simulink model "wind_part"  (R2023b)
settings: Solver=VariableStepAuto  StartTime=0.0  StopTime=5  RelTol=1e-3
InitFcn:
  | Ld=0.3;
  | Lq=0.2;
  | Rs=2;
  | 
  | p=1;
  | Psi=0.2;
  | 
  | J=0.0005;
  | FF=0.0001;
  | 
  | KP_Id=1.28;
  | KI_Id=16.21;
  | KP_Iq=0.94;
  | KI_Iq=4.90;
  | 
  | KP_w=0.0784880455322167;
  | KI_w=0.0288211791619406;
  | 
  | f_pwm=1000;
  | Udc=50;
  | Ns=1;
  | Np=1;
  | R1=0.29;
  | C0=2100;
  | Cv=623;
  | R2=1.92;
  | C2=172;
  | 
  | %data_omega = load('max_CP_omega.mat');
  | 
  | %max_CP_omega = data_omega.max_CP_omega;
  | 
  | %max_CP_omega_param = Simulink.Parameter(max_CP_omega);
  | 
  | %max_CP_omega_param.CoderInfo.StorageClass = 'ExportedGlobal';
libraries: spsMosfetLib x6, simulink x6, slpidlib x4, spsCurrentMeasurementLib x4, spsSeriesRLCBranchLib x3, spsVoltageMeasurementLib x1, spsPermanentMagnetSynchronousMachineLib x1, spsdq0toabcLib x1, spsabctodq0Lib x1, spspowerguiLib x1
settings Model: Creator=hadek  LastModifiedBy=Peter
settings SolverCC: ZeroCrossAlgorithm=Adaptive  AlgebraicLoopSolver=TrustRegion
settings DataIOCC: SaveFormat=StructureWithTime  ReturnWorkspaceOutputs=off
settings DebuggingCC: IgnoredZcDiagnostic=none  UnconnectedInputMsg=warning  UnconnectedOutputMsg=warning  UnconnectedLineMsg=warning  ArithmeticOperatorsInVariantConditions=warning
settings ModelReferenceCC: EnableRefExpFcnMdlSchedulingChecks=on
settings SFSimCC: SimUseLocalCustomCode=off  CustomCodeUndefinedFunction=UseInterfaceOnly
settings RTWCC: RTWUseLocalCustomCode=off

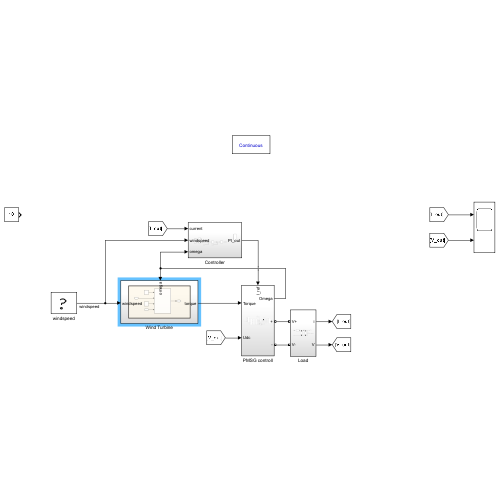
[thumbnail: Simulink's stored preview of the top-level diagram]
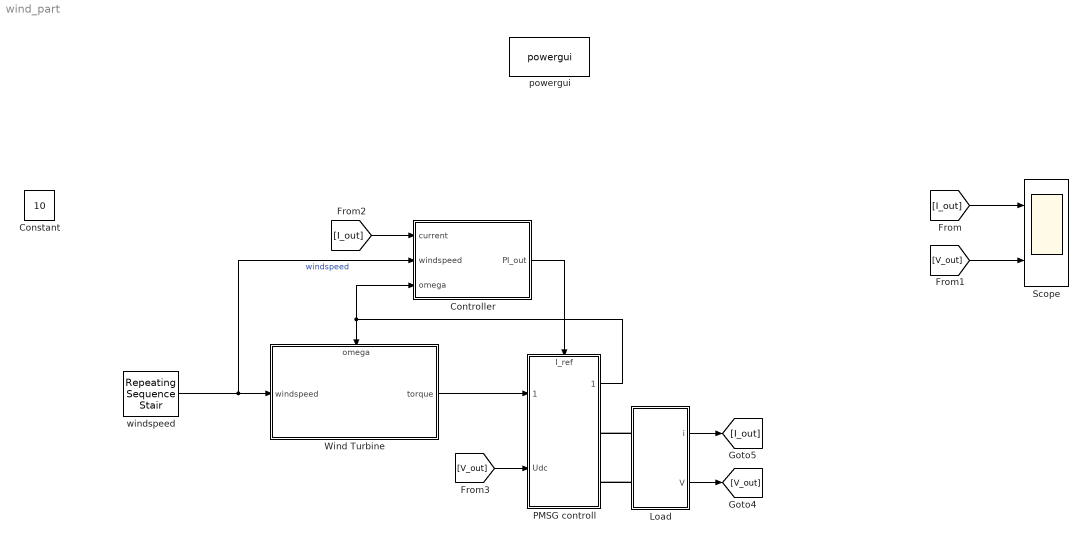
== system wind_part ==
  Constant : Constant  Value=10
  Controller : Subsystem
  Load : Subsystem
  PMSG controll : Subsystem
      settings: PortSchema="{\"entries\":[{\"content\":{\"sides\":[{\"content\":{\"connectorIds\":[\"In1\",\"In2\"]},\"type\":\"ConnectorPlacement.EquallySpacedRectSide\",\"uuid\":\"6ff45732-1fbe-44e6-bbf0-a97c0cfc251c\"},{\"content\":{\"connectorIds\":[\"Out1\",\"RConn1\",\"RConn2\"],\"side\":\"RIGHT\"},\"type\":\"ConnectorPlacement.EquallySpacedRectSide\",\"uuid\":\"615f7fbd-60ca-4bdf-8315-88a0e11d104a\"},{\"content\":{\"connectorIds\":[\"In3\"],\"side\":\"TOP\"},\"type\":\"ConnectorPlacement.EquallySpacedRectSide\",\"uuid\":\"73f43a16-ba4f-4676-a4ee-aa4b37dc4906\"}]},\"type\":\"ConnectorPlacement.EquallySpacedConnector\",\"uuid\":\"b405ac4b-096d-4645-a2b2-df92df1fd96d\"}],\"packageUris\":[\"http://schema.mathworks.com/mf0/Connector/R2020b\"],\"version\":\"1.0\"}"
  Scope : Scope  NumInputPorts=2
  Wind Turbine : Subsystem
      settings: PortSchema="{\"entries\":[{\"content\":{\"sides\":[{\"content\":{\"connectorIds\":[\"In1\"]},\"type\":\"ConnectorPlacement.EquallySpacedRectSide\",\"uuid\":\"d9607854-6c60-486c-bfea-e5bdfd6c8fa9\"},{\"content\":{\"connectorIds\":[\"Out1\"],\"side\":\"RIGHT\"},\"type\":\"ConnectorPlacement.EquallySpacedRectSide\",\"uuid\":\"5fa891cc-5ceb-404b-bebb-ba93c08d2f38\"},{\"content\":{\"connectorIds\":[\"In2\"],\"side\":\"TOP\"},\"type\":\"ConnectorPlacement.EquallySpacedRectSide\",\"uuid\":\"4840ec60-9cf6-480c-919e-88edc7040649\"}]},\"type\":\"ConnectorPlacement.EquallySpacedConnector\",\"uuid\":\"84375009-51d5-45f0-a301-b98d1305d1b8\"}],\"packageUris\":[\"http://schema.mathworks.com/mf0/Connector/R2020b\"],\"version\":\"1.0\"}"
  powergui : spspowerguiLib/powergui  Priority=1  SimulationMode=Continuous  SampleTime=50e-6  frequency=60  Iterations=50  frequencyindice=0  Pbase=100e6  ErrMax=1e-4  UnitsV=kV  UnitsW=MW  buscounter=0  FunctionMessages=off  echomessages=off  EnableUseOfTLC=off  CurrentSourceSwitches=off  DisableSnubberDevices=off  DisableRonSwitches=off  DisableVfSwitches=off  DisplayEquations=off  AutomaticDiscreteSolvers=off  SolverType=Tustin/Backward Euler (TBE)  Interpol=off  ExternalGateDelay=off  methode=off  Ts=100  x0status=blocks  SPID=on  SwTol=0  HookPort=off  NonlinearTolerance=1e-4  nMaxIteration=100  ContinueOnMaxIteration=off  RestoreLinks=warning  ResistiveCurrentMeasurement=off  Frange=[0:2:500]  Ylog=off  Xlog=on  ShowGrid=off  save=off  variable=ZData  structure=0  ZoomFFT=off  StartTime=0.0  cycles=1  DisplayStyle=1  fundamental=60  FreqAxis=off  MaxFrequency=1000  frequencyindicesteady=1  RmsSteady=1  display=off
  windspeed : simulink/Sources/Repeating Sequence Stair  OutValues=windspeed  tsamp=0.2  OutMin=[]  OutMax=[]  OutDataTypeStr=double  OutputDataTypeScalingMode=double  OutDataType=fixdt(0,8)  ConRadixGroup=Best Precision: Vector-wise  OutScaling=2^-12
  wires:
  Load/1(i) -> [I_out]
  Load/2(V) -> [V_out]
  Wind Turbine/1(torque) -> PMSG controll/1(Torque)
  [I_out] -> Scope/1
  [V_out] -> Scope/2
  PMSG controll/1(Omega) -> Controller/3(omega), Wind Turbine/2(omega)
  Controller/1(PI_out) -> PMSG controll/3(I_ref)
  [I_out] -> Controller/1(current)
  [V_out] -> PMSG controll/2(Udc)
  windspeed/1 -> Wind Turbine/1(windspeed), Controller/2(windspeed)  "windspeed"
  connections:
  Load/LConn1 -- PMSG controll/RConn1
  Load/LConn2 -- PMSG controll/RConn2

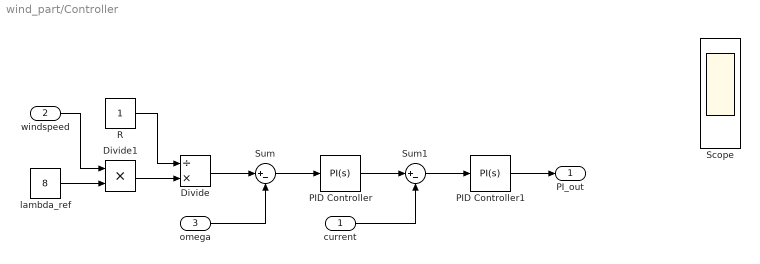
== system wind_part/Controller ==
  current : Inport
  windspeed : Inport  Port=2
  omega : Inport  Port=3
  Divide : Product  Inputs=/*
  Divide1 : Product  Inputs=**
  PID Controller : slpidlib/PID Controller  Controller=PI  Form=Parallel  TimeDomain=Continuous-time  UseExternalTs=off  SampleTime=-1  IntegratorMethod=Forward Euler  FilterMethod=Forward Euler  ControllerParametersSource=internal  P=1  I=1  UseKiTs=off  D=0  N=100  UseFilter=on  TunerSelectOption=Transfer Function Based (PID Tuner App)  InitialConditionSource=internal  InitialConditionForIntegrator=0  InitialConditionForFilter=0  DifferentiatorICPrevScaledInput=0  ExternalReset=none  TrackingMode=off  Kt=1  LimitOutput=off  SatLimitsSource=internal  UpperSaturationLimit=20  LowerSaturationLimit=-20  LinearizeAsGain=on  AntiWindupMode=none  Kb=1  LimitIntegrator=off  UpperIntegratorSaturationLimit=inf  LowerIntegratorSaturationLimit=-inf  POutMin=[]  POutMax=[]  IOutMin=[]  IOutMax=[]  DOutMin=[]  DOutMax=[]  NOutMin=[]  NOutMax=[]  SumOutMin=[]  SumOutMax=[]  SaturationOutMin=[]  SaturationOutMax=[]  PParamMin=[]  PParamMax=[]  IParamMin=[]  IParamMax=[]  DParamMin=[]  DParamMax=[]  NParamMin=[]  NParamMax=[]  KbParamMin=[]  KbParamMax=[]  KtParamMin=[]  KtParamMax=[]  KbOutMin=[]  KbOutMax=[]  KtOutMin=[]  KtOutMax=[]  IntegratorOutMin=[]  IntegratorOutMax=[]  FilterOutMin=[]  FilterOutMax=[]  SumI1OutMin=[]  SumI1OutMax=[]  SumI2OutMin=[]  SumI2OutMax=[]  SumI3OutMin=[]  SumI3OutMax=[]  SumI4OutMin=[]  SumI4OutMax=[]  SumDOutMin=[]  SumDOutMax=[]  DifferentiatorOutMin=[]  DifferentiatorOutMax=[]  FilterDiffOutCoefMin=[]  FilterDiffOutCoefMax=[]  ReciprocalOutMin=[]  ReciprocalOutMax=[]  SumDenOutMin=[]  SumDenOutMax=[]  SumNumOutMin=[]  SumNumOutMax=[]  DivideOutMin=[]  DivideOutMax=[]  UdiffTsProdOutMin=[]  UdiffTsProdOutMax=[]  NTsProdOutMin=[]  NTsProdOutMax=[]  UintegralTsProdOutMin=[]  UintegralTsProdOutMax=[]  UngainTsProdOutMin=[]  UngainTsProdOutMax=[]  ClampingZeroOutDataTypeStr=Inherit: Inherit via back propagation  ClampingZeroOutMin=[]  ClampingZeroOutMax=[]  FilterDenConstantOutDataTypeStr=Inherit: Inherit via back propagation  FilterDenConstantOutMin=[]  FilterDenConstantOutMax=[]  PCopyOutDataTypeStr=Inherit: Inherit via back propagation  PCopyOutMin=[]  PCopyOutMax=[]  NCopyOutDataTypeStr=Inherit: Inherit via back propagation  NCopyOutMin=[]  NCopyOutMax=[]  IntegratorContinuousStateAttributes=''  IntegratorStateMustResolveToSignalObject=off  IntegratorRTWStateStorageClass=Auto  FilterContinuousStateAttributes=''  FilterStateMustResolveToSignalObject=off  FilterRTWStateStorageClass=Auto  ParallelPVariant=InternalParameters  IdealPVariant=Disabled  IVariant=InternalParameters  DVariant=Disabled  IntegratorVariant=Continuous  SatVariant=Disabled  AWVariant=Passthrough  PCopyVariant=Disabled  TRVariant=Disabled  FdbkBlocksVariant=Forward  IdealPFdbkVariant=Disabled  SatFdbkVariant=Disabled  DerivativeFilterVariant=Disabled  NVariant=Disabled  NCopyVariant=Disabled_SignalSpec  FilterICVariant=Disabled  IntegratorICVariant=InternalICs  ExternalResetVariant=Disabled  TRSumVariant=Passthrough  SumFdbkVariant=Disabled  SumVariant=Sum_PI  TsampFilterVariant=InternalTs  TsampNgainVariant=Passthrough  TsampIntegralVariant=Disabled_SignalSpec  ExternalSaturationOutDataTypeStr=Inherit: Same as second input
  PID Controller1 : slpidlib/PID Controller  Controller=PI  Form=Parallel  TimeDomain=Continuous-time  UseExternalTs=off  SampleTime=-1  IntegratorMethod=Forward Euler  FilterMethod=Forward Euler  ControllerParametersSource=internal  P=1  I=1  UseKiTs=off  D=0  N=100  UseFilter=on  TunerSelectOption=Transfer Function Based (PID Tuner App)  InitialConditionSource=internal  InitialConditionForIntegrator=0  InitialConditionForFilter=0  DifferentiatorICPrevScaledInput=0  ExternalReset=none  TrackingMode=off  Kt=1  LimitOutput=off  SatLimitsSource=internal  UpperSaturationLimit=20  LowerSaturationLimit=-20  LinearizeAsGain=on  AntiWindupMode=none  Kb=1  LimitIntegrator=off  UpperIntegratorSaturationLimit=inf  LowerIntegratorSaturationLimit=-inf  POutMin=[]  POutMax=[]  IOutMin=[]  IOutMax=[]  DOutMin=[]  DOutMax=[]  NOutMin=[]  NOutMax=[]  SumOutMin=[]  SumOutMax=[]  SaturationOutMin=[]  SaturationOutMax=[]  PParamMin=[]  PParamMax=[]  IParamMin=[]  IParamMax=[]  DParamMin=[]  DParamMax=[]  NParamMin=[]  NParamMax=[]  KbParamMin=[]  KbParamMax=[]  KtParamMin=[]  KtParamMax=[]  KbOutMin=[]  KbOutMax=[]  KtOutMin=[]  KtOutMax=[]  IntegratorOutMin=[]  IntegratorOutMax=[]  FilterOutMin=[]  FilterOutMax=[]  SumI1OutMin=[]  SumI1OutMax=[]  SumI2OutMin=[]  SumI2OutMax=[]  SumI3OutMin=[]  SumI3OutMax=[]  SumI4OutMin=[]  SumI4OutMax=[]  SumDOutMin=[]  SumDOutMax=[]  DifferentiatorOutMin=[]  DifferentiatorOutMax=[]  FilterDiffOutCoefMin=[]  FilterDiffOutCoefMax=[]  ReciprocalOutMin=[]  ReciprocalOutMax=[]  SumDenOutMin=[]  SumDenOutMax=[]  SumNumOutMin=[]  SumNumOutMax=[]  DivideOutMin=[]  DivideOutMax=[]  UdiffTsProdOutMin=[]  UdiffTsProdOutMax=[]  NTsProdOutMin=[]  NTsProdOutMax=[]  UintegralTsProdOutMin=[]  UintegralTsProdOutMax=[]  UngainTsProdOutMin=[]  UngainTsProdOutMax=[]  ClampingZeroOutDataTypeStr=Inherit: Inherit via back propagation  ClampingZeroOutMin=[]  ClampingZeroOutMax=[]  FilterDenConstantOutDataTypeStr=Inherit: Inherit via back propagation  FilterDenConstantOutMin=[]  FilterDenConstantOutMax=[]  PCopyOutDataTypeStr=Inherit: Inherit via back propagation  PCopyOutMin=[]  PCopyOutMax=[]  NCopyOutDataTypeStr=Inherit: Inherit via back propagation  NCopyOutMin=[]  NCopyOutMax=[]  IntegratorContinuousStateAttributes=''  IntegratorStateMustResolveToSignalObject=off  IntegratorRTWStateStorageClass=Auto  FilterContinuousStateAttributes=''  FilterStateMustResolveToSignalObject=off  FilterRTWStateStorageClass=Auto  ParallelPVariant=InternalParameters  IdealPVariant=Disabled  IVariant=InternalParameters  DVariant=Disabled  IntegratorVariant=Continuous  SatVariant=Disabled  AWVariant=Passthrough  PCopyVariant=Disabled  TRVariant=Disabled  FdbkBlocksVariant=Forward  IdealPFdbkVariant=Disabled  SatFdbkVariant=Disabled  DerivativeFilterVariant=Disabled  NVariant=Disabled  NCopyVariant=Disabled_SignalSpec  FilterICVariant=Disabled  IntegratorICVariant=InternalICs  ExternalResetVariant=Disabled  TRSumVariant=Passthrough  SumFdbkVariant=Disabled  SumVariant=Sum_PI  TsampFilterVariant=InternalTs  TsampNgainVariant=Passthrough  TsampIntegralVariant=Disabled_SignalSpec  ExternalSaturationOutDataTypeStr=Inherit: Same as second input
  R : Constant
  Scope : Scope  NumInputPorts=5
  Sum : Sum  Inputs=|+-
  Sum1 : Sum  Inputs=|+-
  lambda_ref : Constant  Value=8
  PI_out : Outport
  wires:
  R/1 -> Divide/1
  lambda_ref/1 -> Divide1/2
  Divide1/1 -> Divide/2
  windspeed/1 -> Divide1/1
  Sum/1 -> PID Controller/1
  Divide/1 -> Sum/1
  Sum1/1 -> PID Controller1/1
  PID Controller1/1 -> PI_out/1
  PID Controller/1 -> Sum1/1
  current/1 -> Sum1/2
  omega/1 -> Sum/2

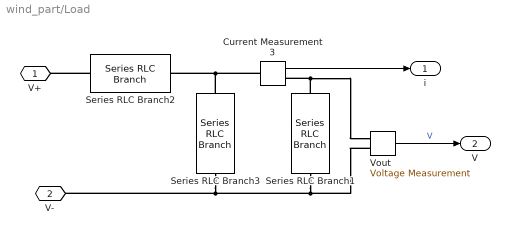
== system wind_part/Load ==
  " Vout" : spsVoltageMeasurementLib/Voltage Measurement  PhasorSimulation=off  OutputType=Complex  PSBequivalent=0
  Current Measurement3 : spsCurrentMeasurementLib/Current Measurement  PhasorSimulation=off  OutputType=Complex  PSBequivalent=0
  Series RLC Branch1 : spsSeriesRLCBranchLib/Series RLC Branch  LConnTagsString=__new0  RConnTagsString=__new0  BranchType=R  Resistance=10  Inductance=1e-3  SetiL0=off  InitialCurrent=0  Capacitance=2e-3  Setx0=off  InitialVoltage=0  Measurements=None
  Series RLC Branch2 : spsSeriesRLCBranchLib/Series RLC Branch  LConnTagsString=__new0  RConnTagsString=__new0  BranchType=L  Resistance=10  Inductance=100e-3  SetiL0=off  InitialCurrent=0  Capacitance=2e-3  Setx0=off  InitialVoltage=0  Measurements=None
  Series RLC Branch3 : spsSeriesRLCBranchLib/Series RLC Branch  LConnTagsString=__new0  RConnTagsString=__new0  BranchType=C  Resistance=10  Inductance=1e-3  SetiL0=off  InitialCurrent=0  Capacitance=2e-3  Setx0=on  InitialVoltage=50  Measurements=None
  V+ : PMIOPort  Side=Left
  V- : PMIOPort  Port=2  Side=Left
  i : Outport
  V : Outport  Port=2
  wires:
  " Vout"/1 -> V/1  "V"
  Current Measurement3/1 -> i/1
  connections:
  Series RLC Branch3/LConn1 -- Current Measurement3/LConn1 -- Series RLC Branch2/RConn1
  Current Measurement3/RConn1 -- Series RLC Branch1/LConn1 -- " Vout"/LConn1
  Series RLC Branch3/RConn1 -- " Vout"/LConn2 -- Series RLC Branch1/RConn1 -- V-/RConn1
  Series RLC Branch2/LConn1 -- V+/RConn1

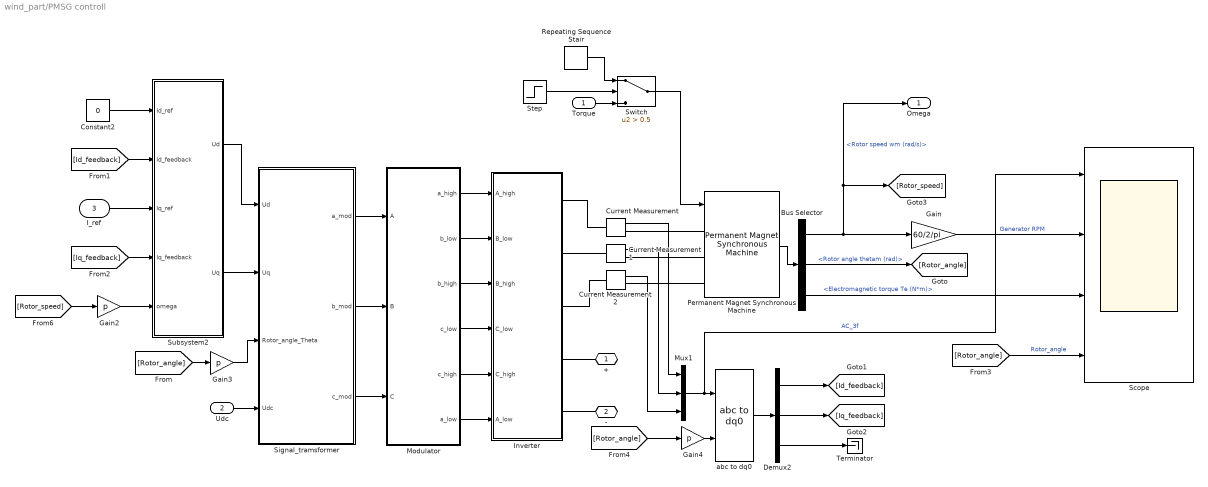
== system wind_part/PMSG controll ==
  Torque : Inport
  Udc : Inport  Port=2
  I_ref : Inport  Port=3
  Bus Selector : BusSelector  OutputSignals=Rotor speed wm (rad/s),Rotor angle thetam (rad),Electromagnetic torque Te (N*m)
  Constant2 : Constant  Value=0
  Current Measurement : spsCurrentMeasurementLib/Current Measurement  PhasorSimulation=off  OutputType=Complex  PSBequivalent=0
  Current Measurement1 : spsCurrentMeasurementLib/Current Measurement  PhasorSimulation=off  OutputType=Complex  PSBequivalent=0
  Current Measurement2 : spsCurrentMeasurementLib/Current Measurement  PhasorSimulation=off  OutputType=Complex  PSBequivalent=0
  Demux2 : Demux  Outputs=3
  Gain : Gain  Gain=60/2/pi
  Gain2 : Gain  Gain=p
  Gain3 : Gain  Gain=p
  Gain4 : Gain  Gain=p
  Inverter : Subsystem
  Modulator : Subsystem
  Mux1 : Mux  Inputs=3
  Permanent Magnet Synchronous Machine : spsPermanentMagnetSynchronousMachineLib/Permanent Magnet Synchronous Machine  NbPhases=3  FluxDistribution=Sinusoidal  RotorType=Salient-pole  MechanicalLoad=Torque Tm  PresetModel=No  ShowDetailedParameters=on  MeasurementBus=off  Resistance=Rs  Inductance=8.5e-3  dqInductances=[Ld,Lq]  La=0.000395  MachineConstant=Flux linkage established by magnets (V.s)  Flux=Psi  VoltageCst=36.276  TorqueCst=0.3  Flat=120  Mechanical=[J FF p 0]  PolePairs=4  InitialConditions=[0,0, 0,0]  InitialConditions5ph=[0 0 0 0 0 0]  RefAngle=90 degrees behind phase A axis (modified Park)  IterativeDiscreteModel=Trapezoidal non iterative  TsBlock=-1  TsPowergui=0
  Repeating Sequence Stair : simulink/Sources/Repeating Sequence Stair  OutValues=0.1:0.1:5  tsamp=0.02  OutMin=[]  OutMax=[]  OutDataTypeStr=double  OutputDataTypeScalingMode=double  OutDataType=fixdt(0,8)  ConRadixGroup=Best Precision: Vector-wise  OutScaling=2^-12
  Scope : Scope  NumInputPorts=4
  Signal_tramsformer : Subsystem
  Step : Step  Time=5  Before=1  After=0  SampleTime=0
  Subsystem2 : Subsystem
  Switch : Switch  Criteria=u2 > Threshold  Threshold=0.5  SaturateOnIntegerOverflow=off  InputSameDT=off
  Terminator : Terminator
  abc to dq0 : spsabctodq0Lib/abc to dq0  Alignment=90 degrees behind phase A axis
  + : PMIOPort  Side=Right
  - : PMIOPort  Port=2  Side=Right
  Omega : Outport
  wires:
  Current Measurement/1 -> Mux1/1
  [Rotor_speed] -> Gain2/1
  [Rotor_angle] -> Gain4/1
  Current Measurement2/1 -> Mux1/3
  [Rotor_angle] -> Gain3/1
  Subsystem2/2(Uq) -> Signal_tramsformer/2(Uq)
  Demux2/2 -> [Iq_feedback]
  Bus Selector/1 -> [Rotor_speed], Omega/1, Gain/1  "<Rotor speed wm (rad/s)>"
  [Id_feedback] -> Subsystem2/2(Id_feedback)
  Signal_tramsformer/3(c_mod) -> Modulator/3(C)
  Bus Selector/3 -> Scope/3  "<Electromagnetic torque Te (N*m)>"
  Bus Selector/2 -> [Rotor_angle]  "<Rotor angle thetam (rad)>"
  abc to dq0/1 -> Demux2/1
  Demux2/1 -> [Id_feedback]
  Signal_tramsformer/2(b_mod) -> Modulator/2(B)
  Constant2/1 -> Subsystem2/1(Id_ref)
  Mux1/1 -> Scope/1, abc to dq0/1  "AC_3f"
  Demux2/3 -> Terminator/1
  Current Measurement1/1 -> Mux1/2
  [Iq_feedback] -> Subsystem2/4(Iq_feedback)
  Gain/1 -> Scope/2  "Generator RPM"
  Signal_tramsformer/1(a_mod) -> Modulator/1(A)
  I_ref/1 -> Subsystem2/3(Iq_ref)
  Subsystem2/1(Ud) -> Signal_tramsformer/1(Ud)
  [Rotor_angle] -> Scope/4  "Rotor_angle"
  Permanent Magnet Synchronous Machine/1 -> Bus Selector/1
  Gain4/1 -> abc to dq0/2
  Gain3/1 -> Signal_tramsformer/3(Rotor_angle_Theta)
  Gain2/1 -> Subsystem2/5(omega)
  Torque/1 -> Switch/3
  Udc/1 -> Signal_tramsformer/4(Udc)
  Modulator/5(c_high) -> Inverter/5(C_high)
  Modulator/6(a_low) -> Inverter/6(A_low)
  Modulator/4(c_low) -> Inverter/4(C_low)
  Modulator/2(b_low) -> Inverter/2(B_low)
  Modulator/1(a_high) -> Inverter/1(A_high)
  Modulator/3(b_high) -> Inverter/3(" B_high")
  Step/1 -> Switch/2
  Switch/1 -> Permanent Magnet Synchronous Machine/1
  Repeating Sequence Stair/1 -> Switch/1
  connections:
  Current Measurement2/RConn1 -- Permanent Magnet Synchronous Machine/LConn3
  Current Measurement1/RConn1 -- Permanent Magnet Synchronous Machine/LConn2
  Inverter/RConn3 -- Current Measurement2/LConn1
  Inverter/RConn1 -- Current Measurement/LConn1
  Inverter/RConn2 -- Current Measurement1/LConn1
  Permanent Magnet Synchronous Machine/LConn1 -- Current Measurement/RConn1
  Inverter/RConn5 -- -/RConn1
  Inverter/RConn4 -- +/RConn1

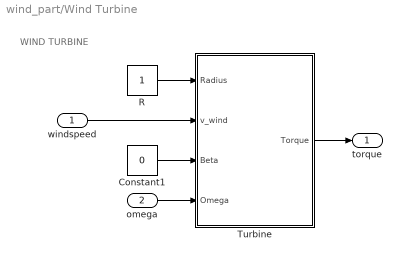
== system wind_part/Wind Turbine ==
  note: WIND TURBINE
  windspeed : Inport
  omega : Inport  Port=2
  Constant1 : Constant  Value=0
  R : Constant
  Turbine : Subsystem
  torque : Outport
  wires:
  R/1 -> Turbine/1(Radius)
  omega/1 -> Turbine/4(Omega)
  Constant1/1 -> Turbine/3(Beta)
  windspeed/1 -> Turbine/2(v_wind)
  Turbine/1(Torque) -> torque/1

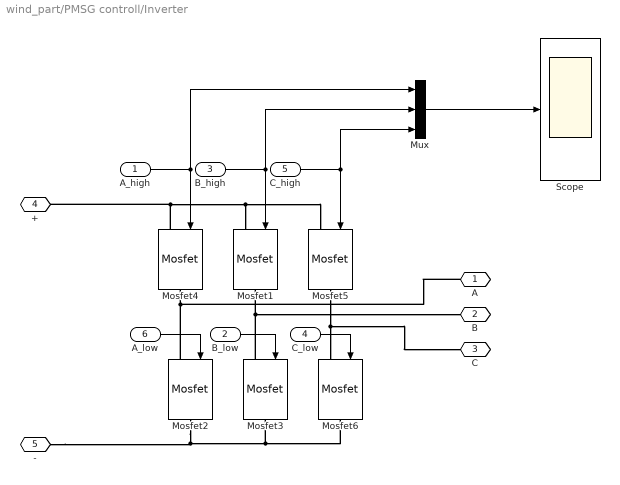
== system wind_part/PMSG controll/Inverter ==
  A_high : Inport
  B_low : Inport  Port=2
  " B_high" : Inport  Port=3
  C_low : Inport  Port=4
  C_high : Inport  Port=5
  A_low : Inport  Port=6
  Mosfet{1..6} (6 alike) : spsMosfetLib/Mosfet  Ron=0.1  Lon=0  Rd=0.01  Vfd=0  IC=0  Rs=1e5  Cs=inf  Measurements=off
  Mux : Mux  Inputs=3
  Scope : Scope
  A : PMIOPort  Side=Right
  B : PMIOPort  Port=2  Side=Right
  C : PMIOPort  Port=3  Side=Right
  + : PMIOPort  Port=4  Side=Right
  - : PMIOPort  Port=5  Side=Right
  wires:
  A_high/1 -> Mux/1, Mosfet4/1
  C_high/1 -> Mux/3, Mosfet5/1
  " B_high"/1 -> Mux/2, Mosfet1/1
  Mux/1 -> Scope/1
  B_low/1 -> Mosfet3/1
  C_low/1 -> Mosfet6/1
  A_low/1 -> Mosfet2/1
  connections:
  Mosfet4/LConn1 -- +/RConn1 -- Mosfet5/LConn1 -- Mosfet1/LConn1
  Mosfet5/RConn1 -- Mosfet6/LConn1 -- C/RConn1
  Mosfet3/LConn1 -- B/RConn1 -- Mosfet1/RConn1
  Mosfet2/RConn1 -- -/RConn1 -- Mosfet6/RConn1 -- Mosfet3/RConn1
  Mosfet2/LConn1 -- A/RConn1 -- Mosfet4/RConn1

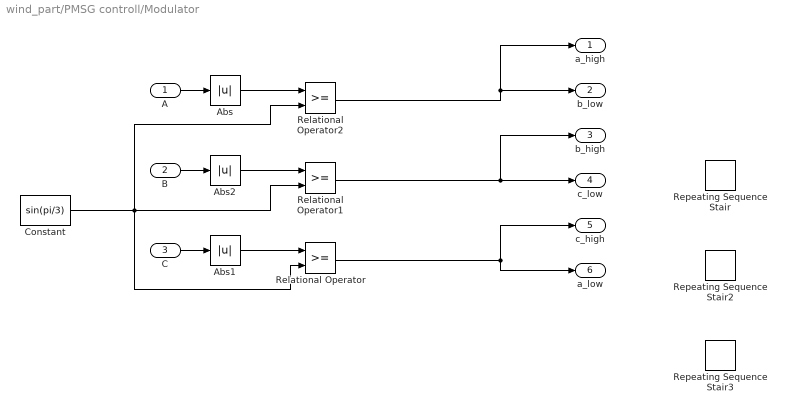
== system wind_part/PMSG controll/Modulator ==
  A : Inport
  B : Inport  Port=2
  C : Inport  Port=3
  Abs : Abs  SaturateOnIntegerOverflow=off
  Abs1 : Abs  SaturateOnIntegerOverflow=off
  Abs2 : Abs  SaturateOnIntegerOverflow=off
  Constant : Constant  Value=sin(pi/3)
  Relational Operator : RelationalOperator  OutDataTypeStr=boolean  RndMeth=Simplest  InputSameDT=off
  Relational Operator1 : RelationalOperator  OutDataTypeStr=boolean  RndMeth=Simplest  InputSameDT=off
  Relational Operator2 : RelationalOperator  OutDataTypeStr=boolean  RndMeth=Simplest  InputSameDT=off
  Repeating Sequence Stair : simulink/Sources/Repeating Sequence Stair  OutValues=[0 1 1 0 0 0 0 1 1 0 0 0]  tsamp=30/(360)  OutMin=[]  OutMax=[]  OutDataTypeStr=double  OutputDataTypeScalingMode=double  OutDataType=fixdt(0,8)  ConRadixGroup=Best Precision: Vector-wise  OutScaling=2^-12
  Repeating Sequence Stair2 : simulink/Sources/Repeating Sequence Stair  OutValues=[1 0 0 0 0 1 1 0 0 0 0 1]  tsamp=30/360  OutMin=[]  OutMax=[]  OutDataTypeStr=double  OutputDataTypeScalingMode=double  OutDataType=fixdt(0,8)  ConRadixGroup=Best Precision: Vector-wise  OutScaling=2^-12
  Repeating Sequence Stair3 : simulink/Sources/Repeating Sequence Stair  OutValues=[0 0 0 1 1 0 0 0 0 1 1 0]  tsamp=30/360  OutMin=[]  OutMax=[]  OutDataTypeStr=double  OutputDataTypeScalingMode=double  OutDataType=fixdt(0,8)  ConRadixGroup=Best Precision: Vector-wise  OutScaling=2^-12
  a_high : Outport
  b_low : Outport  Port=2
  b_high : Outport  Port=3
  c_low : Outport  Port=4
  c_high : Outport  Port=5
  a_low : Outport  Port=6
  wires:
  B/1 -> Abs2/1
  C/1 -> Abs1/1
  A/1 -> Abs/1
  Relational Operator2/1 -> a_high/1, b_low/1
  Relational Operator1/1 -> b_high/1, c_low/1
  Relational Operator/1 -> c_high/1, a_low/1
  Constant/1 -> Relational Operator2/2, Relational Operator1/2, Relational Operator/2
  Abs/1 -> Relational Operator2/1
  Abs1/1 -> Relational Operator/1
  Abs2/1 -> Relational Operator1/1

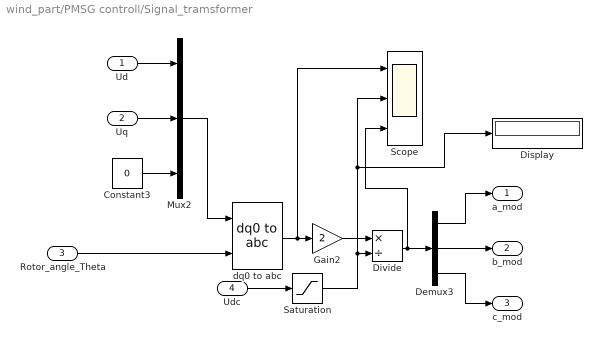
== system wind_part/PMSG controll/Signal_tramsformer ==
  Ud : Inport
  Uq : Inport  Port=2
  Rotor_angle_Theta : Inport  Port=3
  Udc : Inport  Port=4
  Constant3 : Constant  Value=0
  Demux3 : Demux  Outputs=3
  Display : Display
  Divide : Product  Inputs=*/
  Gain2 : Gain  Gain=2
  Mux2 : Mux  Inputs=3
  Saturation : Saturate  UpperLimit=inf  LowerLimit=1e-1
  Scope : Scope  NumInputPorts=3
  dq0 to abc : spsdq0toabcLib/dq0 to abc  Alignment=90 degrees behind phase A axis
  a_mod : Outport
  b_mod : Outport  Port=2
  c_mod : Outport  Port=3
  wires:
  Demux3/1 -> a_mod/1
  Udc/1 -> Saturation/1
  Divide/1 -> Scope/3, Demux3/1
  dq0 to abc/1 -> Scope/1, Gain2/1
  Gain2/1 -> Divide/1
  Mux2/1 -> dq0 to abc/1
  Constant3/1 -> Mux2/3
  Demux3/3 -> c_mod/1
  Demux3/2 -> b_mod/1
  Ud/1 -> Mux2/1
  Uq/1 -> Mux2/2
  Rotor_angle_Theta/1 -> dq0 to abc/2
  Saturation/1 -> Scope/2, Display/1, Divide/2

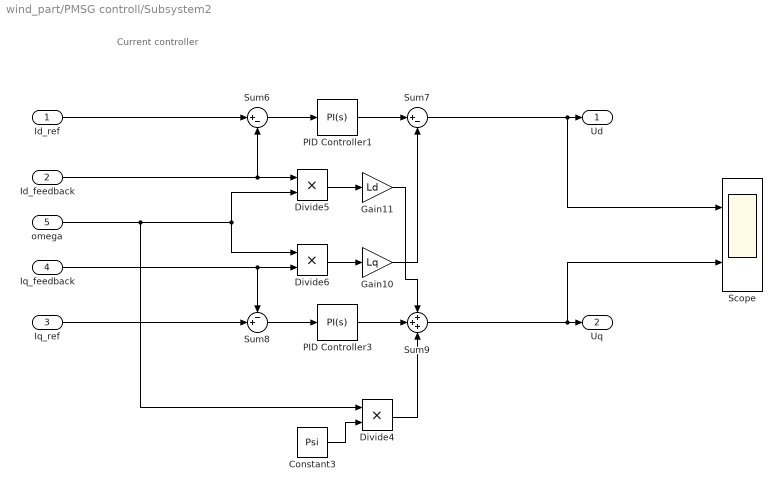
== system wind_part/PMSG controll/Subsystem2 ==
  note: Current controller
  Id_ref : Inport
  Id_feedback : Inport  Port=2
  Iq_ref : Inport  Port=3
  Iq_feedback : Inport  Port=4
  omega : Inport  Port=5
  Constant3 : Constant  Value=Psi
  Divide4 : Product  Inputs=**
  Divide5 : Product  Inputs=**
  Divide6 : Product  Inputs=**
  Gain10 : Gain  Gain=Lq
  Gain11 : Gain  Gain=Ld
  PID Controller1 : slpidlib/PID Controller  Controller=PI  Form=Parallel  TimeDomain=Continuous-time  UseExternalTs=off  SampleTime=-1  IntegratorMethod=Forward Euler  FilterMethod=Forward Euler  ControllerParametersSource=internal  P=KP_Id  I=KI_Id  UseKiTs=off  D=0  N=100  UseFilter=on  TunerSelectOption=Transfer Function Based (PID Tuner App)  InitialConditionSource=internal  InitialConditionForIntegrator=0  InitialConditionForFilter=0  DifferentiatorICPrevScaledInput=0  ExternalReset=none  TrackingMode=off  Kt=1  LimitOutput=off  SatLimitsSource=internal  UpperSaturationLimit=650  LowerSaturationLimit=-650  LinearizeAsGain=on  AntiWindupMode=none  Kb=1  LimitIntegrator=off  UpperIntegratorSaturationLimit=inf  LowerIntegratorSaturationLimit=-inf  POutMin=[]  POutMax=[]  IOutMin=[]  IOutMax=[]  DOutMin=[]  DOutMax=[]  NOutMin=[]  NOutMax=[]  SumOutMin=[]  SumOutMax=[]  SaturationOutMin=[]  SaturationOutMax=[]  PParamMin=[]  PParamMax=[]  IParamMin=[]  IParamMax=[]  DParamMin=[]  DParamMax=[]  NParamMin=[]  NParamMax=[]  KbParamMin=[]  KbParamMax=[]  KtParamMin=[]  KtParamMax=[]  KbOutMin=[]  KbOutMax=[]  KtOutMin=[]  KtOutMax=[]  IntegratorOutMin=[]  IntegratorOutMax=[]  FilterOutMin=[]  FilterOutMax=[]  SumI1OutMin=[]  SumI1OutMax=[]  SumI2OutMin=[]  SumI2OutMax=[]  SumI3OutMin=[]  SumI3OutMax=[]  SumI4OutMin=[]  SumI4OutMax=[]  SumDOutMin=[]  SumDOutMax=[]  DifferentiatorOutMin=[]  DifferentiatorOutMax=[]  FilterDiffOutCoefMin=[]  FilterDiffOutCoefMax=[]  ReciprocalOutMin=[]  ReciprocalOutMax=[]  SumDenOutMin=[]  SumDenOutMax=[]  SumNumOutMin=[]  SumNumOutMax=[]  DivideOutMin=[]  DivideOutMax=[]  UdiffTsProdOutMin=[]  UdiffTsProdOutMax=[]  NTsProdOutMin=[]  NTsProdOutMax=[]  UintegralTsProdOutMin=[]  UintegralTsProdOutMax=[]  UngainTsProdOutMin=[]  UngainTsProdOutMax=[]  ClampingZeroOutDataTypeStr=Inherit: Inherit via back propagation  ClampingZeroOutMin=[]  ClampingZeroOutMax=[]  FilterDenConstantOutDataTypeStr=Inherit: Inherit via back propagation  FilterDenConstantOutMin=[]  FilterDenConstantOutMax=[]  PCopyOutDataTypeStr=Inherit: Inherit via back propagation  PCopyOutMin=[]  PCopyOutMax=[]  NCopyOutDataTypeStr=Inherit: Inherit via back propagation  NCopyOutMin=[]  NCopyOutMax=[]  IntegratorContinuousStateAttributes=''  IntegratorStateMustResolveToSignalObject=off  IntegratorRTWStateStorageClass=Auto  FilterContinuousStateAttributes=''  FilterStateMustResolveToSignalObject=off  FilterRTWStateStorageClass=Auto  ParallelPVariant=InternalParameters  IdealPVariant=Disabled  IVariant=InternalParameters  DVariant=Disabled  IntegratorVariant=Continuous  SatVariant=Disabled  AWVariant=Passthrough  PCopyVariant=Disabled  TRVariant=Disabled  FdbkBlocksVariant=Forward  IdealPFdbkVariant=Disabled  SatFdbkVariant=Disabled  DerivativeFilterVariant=Disabled  NVariant=Disabled  NCopyVariant=Disabled_SignalSpec  FilterICVariant=Disabled  IntegratorICVariant=InternalICs  ExternalResetVariant=Disabled  TRSumVariant=Passthrough  SumFdbkVariant=Disabled  SumVariant=Sum_PI  TsampFilterVariant=InternalTs  TsampNgainVariant=Passthrough  TsampIntegralVariant=Disabled_SignalSpec  ExternalSaturationOutDataTypeStr=Inherit: Same as second input
  PID Controller3 : slpidlib/PID Controller  Controller=PI  Form=Parallel  TimeDomain=Continuous-time  UseExternalTs=off  SampleTime=-1  IntegratorMethod=Forward Euler  FilterMethod=Forward Euler  ControllerParametersSource=internal  P=KP_Iq  I=KI_Iq  UseKiTs=off  D=0  N=100  UseFilter=on  TunerSelectOption=Transfer Function Based (PID Tuner App)  InitialConditionSource=internal  InitialConditionForIntegrator=0  InitialConditionForFilter=0  DifferentiatorICPrevScaledInput=0  ExternalReset=none  TrackingMode=off  Kt=1  LimitOutput=off  SatLimitsSource=internal  UpperSaturationLimit=650  LowerSaturationLimit=-650  LinearizeAsGain=on  AntiWindupMode=none  Kb=1  LimitIntegrator=off  UpperIntegratorSaturationLimit=inf  LowerIntegratorSaturationLimit=-inf  POutMin=[]  POutMax=[]  IOutMin=[]  IOutMax=[]  DOutMin=[]  DOutMax=[]  NOutMin=[]  NOutMax=[]  SumOutMin=[]  SumOutMax=[]  SaturationOutMin=[]  SaturationOutMax=[]  PParamMin=[]  PParamMax=[]  IParamMin=[]  IParamMax=[]  DParamMin=[]  DParamMax=[]  NParamMin=[]  NParamMax=[]  KbParamMin=[]  KbParamMax=[]  KtParamMin=[]  KtParamMax=[]  KbOutMin=[]  KbOutMax=[]  KtOutMin=[]  KtOutMax=[]  IntegratorOutMin=[]  IntegratorOutMax=[]  FilterOutMin=[]  FilterOutMax=[]  SumI1OutMin=[]  SumI1OutMax=[]  SumI2OutMin=[]  SumI2OutMax=[]  SumI3OutMin=[]  SumI3OutMax=[]  SumI4OutMin=[]  SumI4OutMax=[]  SumDOutMin=[]  SumDOutMax=[]  DifferentiatorOutMin=[]  DifferentiatorOutMax=[]  FilterDiffOutCoefMin=[]  FilterDiffOutCoefMax=[]  ReciprocalOutMin=[]  ReciprocalOutMax=[]  SumDenOutMin=[]  SumDenOutMax=[]  SumNumOutMin=[]  SumNumOutMax=[]  DivideOutMin=[]  DivideOutMax=[]  UdiffTsProdOutMin=[]  UdiffTsProdOutMax=[]  NTsProdOutMin=[]  NTsProdOutMax=[]  UintegralTsProdOutMin=[]  UintegralTsProdOutMax=[]  UngainTsProdOutMin=[]  UngainTsProdOutMax=[]  ClampingZeroOutDataTypeStr=Inherit: Inherit via back propagation  ClampingZeroOutMin=[]  ClampingZeroOutMax=[]  FilterDenConstantOutDataTypeStr=Inherit: Inherit via back propagation  FilterDenConstantOutMin=[]  FilterDenConstantOutMax=[]  PCopyOutDataTypeStr=Inherit: Inherit via back propagation  PCopyOutMin=[]  PCopyOutMax=[]  NCopyOutDataTypeStr=Inherit: Inherit via back propagation  NCopyOutMin=[]  NCopyOutMax=[]  IntegratorContinuousStateAttributes=''  IntegratorStateMustResolveToSignalObject=off  IntegratorRTWStateStorageClass=Auto  FilterContinuousStateAttributes=''  FilterStateMustResolveToSignalObject=off  FilterRTWStateStorageClass=Auto  ParallelPVariant=InternalParameters  IdealPVariant=Disabled  IVariant=InternalParameters  DVariant=Disabled  IntegratorVariant=Continuous  SatVariant=Disabled  AWVariant=Passthrough  PCopyVariant=Disabled  TRVariant=Disabled  FdbkBlocksVariant=Forward  IdealPFdbkVariant=Disabled  SatFdbkVariant=Disabled  DerivativeFilterVariant=Disabled  NVariant=Disabled  NCopyVariant=Disabled_SignalSpec  FilterICVariant=Disabled  IntegratorICVariant=InternalICs  ExternalResetVariant=Disabled  TRSumVariant=Passthrough  SumFdbkVariant=Disabled  SumVariant=Sum_PI  TsampFilterVariant=InternalTs  TsampNgainVariant=Passthrough  TsampIntegralVariant=Disabled_SignalSpec  ExternalSaturationOutDataTypeStr=Inherit: Same as second input
  Scope : Scope  NumInputPorts=2
  Sum6 : Sum  Inputs=|+-
  Sum7 : Sum  Inputs=|+-
  Sum8 : Sum  Inputs=-+|
  Sum9 : Sum  Inputs=+++
  Ud : Outport
  Uq : Outport  Port=2
  wires:
  Gain10/1 -> Sum7/2
  PID Controller1/1 -> Sum7/1
  omega/1 -> Divide4/1, Divide6/1, Divide5/2
  Sum6/1 -> PID Controller1/1
  Sum7/1 -> Scope/1, Ud/1
  Sum9/1 -> Scope/2, Uq/1
  Constant3/1 -> Divide4/2
  Divide6/1 -> Gain10/1
  Sum8/1 -> PID Controller3/1
  Divide5/1 -> Gain11/1
  PID Controller3/1 -> Sum9/2
  Divide4/1 -> Sum9/3
  Gain11/1 -> Sum9/1
  Id_ref/1 -> Sum6/1
  Id_feedback/1 -> Divide5/1, Sum6/2
  Iq_ref/1 -> Sum8/2
  Iq_feedback/1 -> Sum8/1, Divide6/2

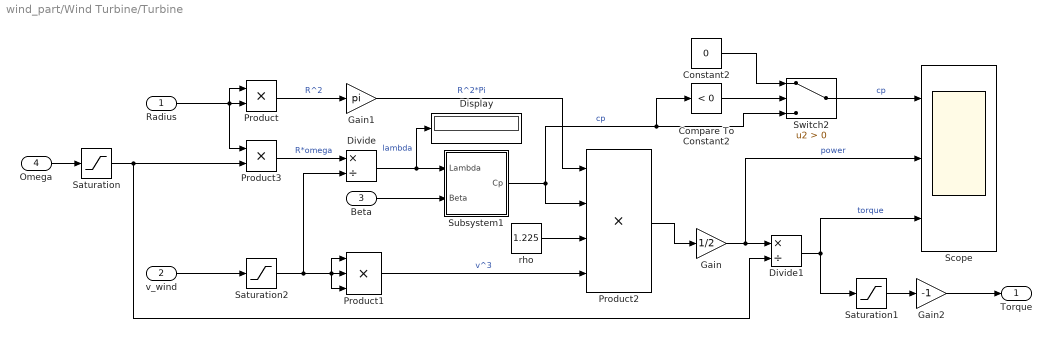
== system wind_part/Wind Turbine/Turbine ==
  Radius : Inport
  v_wind : Inport  Port=2
  Beta : Inport  Port=3
  Omega : Inport  Port=4
  Compare To Constant2 : simulink/Logic and Bit Operations/Compare To Constant  relop=<  const=0  OutDataTypeStr=boolean
  Constant2 : Constant  Value=0
  Display : Display
  Divide : Product  Inputs=*/
  Divide1 : Product  Inputs=*/
  Gain : Gain  Gain=1/2
  Gain1 : Gain  Gain=pi
  Gain2 : Gain  Gain=-1
  Product : Product
  Product1 : Product  Inputs=3
  Product2 : Product  Inputs=4
  Product3 : Product
  Saturation : Saturate  UpperLimit=inf  LowerLimit=1e-6
  Saturation1 : Saturate  UpperLimit=inf  LowerLimit=0
  Saturation2 : Saturate  UpperLimit=inf  LowerLimit=1e-6
  Scope : Scope  NumInputPorts=3
  Subsystem1 : Subsystem
  Switch2 : Switch  Criteria=u2 > Threshold  SaturateOnIntegerOverflow=off  InputSameDT=off
  rho : Constant  Value=1.225
  Torque : Outport  VectorParamsAs1DForOutWhenUnconnected=off
  wires:
  Divide1/1 -> Saturation1/1, Scope/3  "torque"
  Subsystem1/1(Cp) -> Product2/2, Compare To Constant2/1, Switch2/3  "cp"
  Gain1/1 -> Product2/1  "R^2*Pi"
  Beta/1 -> Subsystem1/2(Beta)
  v_wind/1 -> Saturation2/1
  Product/1 -> Gain1/1  "R^2"
  Product2/1 -> Gain/1
  Product1/1 -> Product2/4  "v^3"
  rho/1 -> Product2/3
  Gain/1 -> Divide1/1, Scope/2  "power"
  Constant2/1 -> Switch2/1
  Compare To Constant2/1 -> Switch2/2
  Switch2/1 -> Scope/1  "cp"
  Radius/1 -> Product/1, Product3/1, Product/2
  Product3/1 -> Divide/1  "R*omega"
  Divide/1 -> Display/1, Subsystem1/1(Lambda)  "lambda"
  Omega/1 -> Saturation/1
  Saturation/1 -> Divide1/2, Product3/2
  Saturation1/1 -> Gain2/1
  Gain2/1 -> Torque/1
  Saturation2/1 -> Divide/2, Product1/3, Product1/1, Product1/2

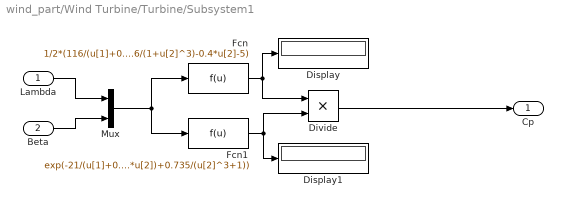
== system wind_part/Wind Turbine/Turbine/Subsystem1 ==
  Lambda : Inport
  Beta : Inport  Port=2
  Display : Display
  Display1 : Display
  Divide : Product  Inputs=**
  Fcn : Fcn  Expr=1/2*(116/(u[1]+0.08*u[2])-4.06/(1+u[2]^3)-0.4*u[2]-5)
  Fcn1 : Fcn  Expr=exp(-21/(u[1]+0.08*u[2])+0.735/(u[2]^3+1))
  Mux : Mux  Inputs=2
  Cp : Outport
  wires:
  Fcn1/1 -> Display1/1, Divide/2
  Fcn/1 -> Display/1, Divide/1
  Divide/1 -> Cp/1
  Mux/1 -> Fcn1/1, Fcn/1
  Beta/1 -> Mux/2
  Lambda/1 -> Mux/1
